simulink model "main"  (R2025b)
settings: Solver=FixedStepAuto  StartTime=0.0  StopTime=25  FixedStep=0.001  RelTol=1e-3
values from neighbouring files (symbols this model uses):
  Fin_MaxAngle = 8    [data.m]
  Physics_Gravity = -9.81    [data.m]
  Physics_SensorsNoiseFactor = 0.5    [data.m]
  PID_DCoeff = 50    [data.m]
  PID_DeadZone = 0.0    (= 0)    [data.m]
  PID_Kd = 50    [data.m]
  PID_Ki = 0    [data.m]
  PID_Kp = 400    [data.m]
  PID_SampleTime = 0.01    [data.m]
  PID_ServoDelay = 0.01    [data.m]
  PID_ServoMaxRate = 400    [data.m]
  Rocket_DesiredRotation = 90    [data.m]
libraries: simulink x5, simulink_extras x2, slpidlib x1, aerolibatmos2 x1, aerolibasang x1, aerolibnav x1, aerolibanim x1
settings Model: Creator=Filip  LastModifiedBy=Filip
settings SolverCC: EnableFixedStepZeroCrossing=on
settings RTWCC: GenCodeOnly=on
settings SimscapeCC: SimscapeLogDecimation=1  SimscapeLogDataHistory=5000

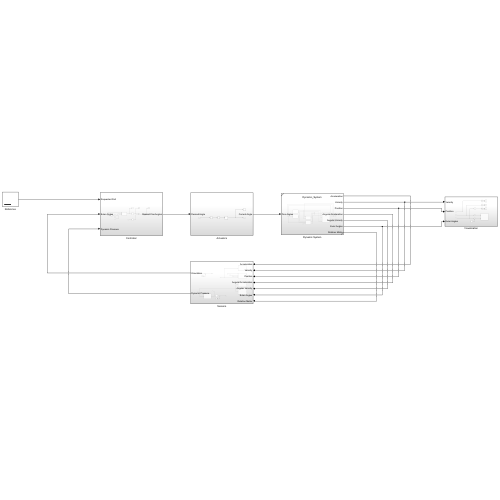
[thumbnail: Simulink's stored preview of the top-level diagram]
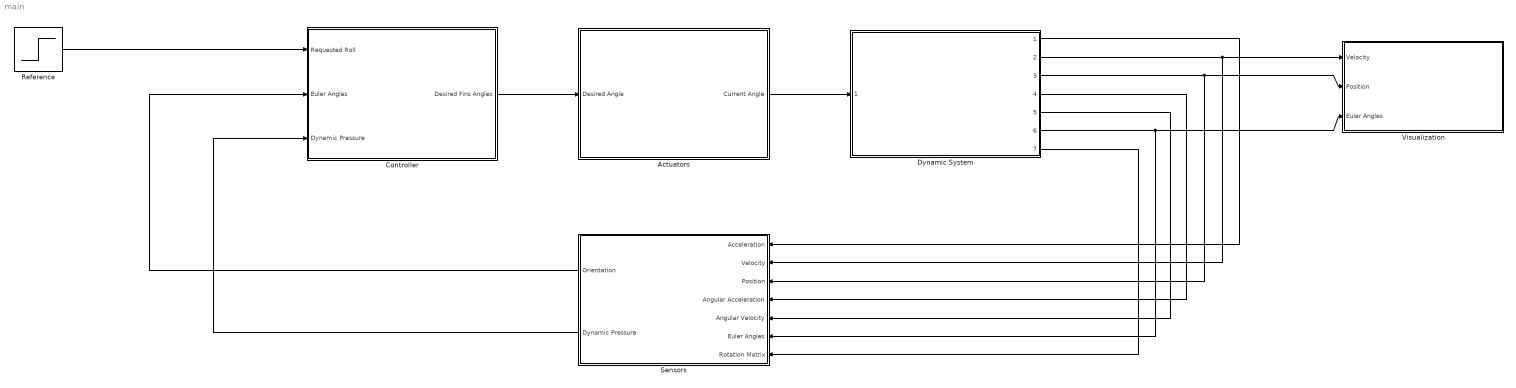
== system main ==
  Actuators : Subsystem
  Controller : Subsystem
  Dynamic System : Subsystem  ReferencedSubsystem=Dynamic_System
  Reference : Step  Time=2  After=Rocket_DesiredRotation  SampleTime=0
  Sensors : Subsystem
  Visualization : Subsystem
  wires:
  Controller/1(Desired Fins Angles) -> Actuators/1(Desired Angle)
  Actuators/1(Current Angle) -> Dynamic System/1
  Reference/1 -> Controller/1(Requested Roll)
  Dynamic System/2 -> Sensors/2(Velocity), Visualization/1(Velocity)
  Dynamic System/3 -> Sensors/3(Position), Visualization/2(Position)
  Dynamic System/6 -> Sensors/6(Euler Angles), Visualization/3(Euler Angles)
  Sensors/1(Orientation) -> Controller/2(Euler Angles)
  Sensors/2(Dynamic Pressure) -> Controller/3(Dynamic Pressure)
  Dynamic System/1 -> Sensors/1(Acceleration)
  Dynamic System/4 -> Sensors/4(Angular Acceleration)
  Dynamic System/5 -> Sensors/5(Angular Velocity)
  Dynamic System/7 -> Sensors/7(Rotation Matrix)

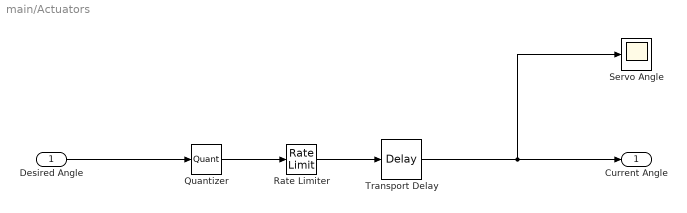
== system main/Actuators ==
  Desired Angle : Inport
  Quantizer : Quantizer  QuantizationInterval=PID_ServoStep
  Rate Limiter : RateLimiter  RisingSlewLimit=+PID_ServoMaxRate  FallingSlewLimit=-PID_ServoMaxRate  SampleTimeMode=inherited
  Servo Angle : Scope
      settings: DataLoggingVariableName=ScopeData2
  Transport Delay : TransportDelay  DelayTime=PID_ServoDelay
  Current Angle : Outport
  wires:
  Rate Limiter/1 -> Transport Delay/1
  Transport Delay/1 -> Servo Angle/1, Current Angle/1
  Quantizer/1 -> Rate Limiter/1
  Desired Angle/1 -> Quantizer/1

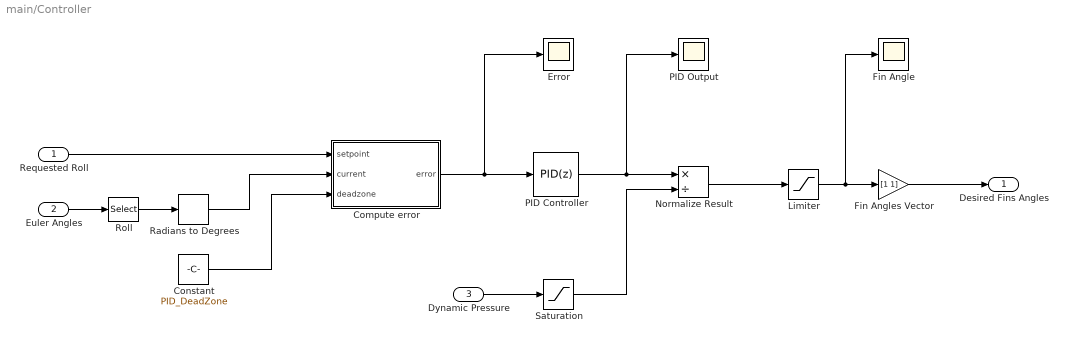
== system main/Controller ==
  Requested Roll : Inport
  Euler Angles : Inport  Port=2
  Dynamic Pressure : Inport  Port=3
  Compute error : MATLAB Function  TreatAsAtomicUnit=on
  Constant : Constant  Value=PID_DeadZone
  Error : Scope
      settings: ActiveDisplayYMinimum=-22.0959398024316  ActiveDisplayYMaximum=103.3390551975684
  Fin Angle : Scope
      settings: DataLoggingVariableName=ScopeData3
  Fin Angles Vector : Gain  Gain=[1 1]
  Limiter : Saturate  UpperLimit=+Fin_MaxAngle  LowerLimit=-Fin_MaxAngle
  Normalize Result : Product  Inputs=*/
  PID Controller : slpidlib/PID Controller  Controller=PID  Form=Parallel  TimeDomain=Discrete-time  UseExternalTs=off  SampleTime=PID_SampleTime  IntegratorMethod=Forward Euler  FilterMethod=Forward Euler  ControllerParametersSource=internal  P=PID_Kp  I=PID_Ki  UseKiTs=off  D=PID_Kd  UseExternalDerivativeSource=off  N=PID_DCoeff  UseFilter=on  TunerSelectOption=Transfer Function Based (PID Tuner App)  InitialConditionSource=internal  InitialConditionForIntegrator=0  InitialConditionForFilter=0  DifferentiatorICPrevScaledInput=0  ExternalReset=none  TrackingMode=off  Kt=1  LimitOutput=off  SatLimitsSource=internal  UpperSaturationLimit=inf  LowerSaturationLimit=-inf  LinearizeAsGain=on  AntiWindupMode=none  Kb=1  LimitIntegrator=off  UpperIntegratorSaturationLimit=inf  LowerIntegratorSaturationLimit=-inf  POutMin=[]  POutMax=[]  IOutMin=[]  IOutMax=[]  DOutMin=[]  DOutMax=[]  NOutMin=[]  NOutMax=[]  SumOutMin=[]  SumOutMax=[]  SaturationOutMin=[]  SaturationOutMax=[]  PParamMin=[]  PParamMax=[]  IParamMin=[]  IParamMax=[]  DParamMin=[]  DParamMax=[]  NParamMin=[]  NParamMax=[]  KbParamMin=[]  KbParamMax=[]  KtParamMin=[]  KtParamMax=[]  KbOutMin=[]  KbOutMax=[]  KtOutMin=[]  KtOutMax=[]  IntegratorOutMin=[]  IntegratorOutMax=[]  FilterOutMin=[]  FilterOutMax=[]  SumI1OutMin=[]  SumI1OutMax=[]  SumI2OutMin=[]  SumI2OutMax=[]  SumI3OutMin=[]  SumI3OutMax=[]  SumI4OutMin=[]  SumI4OutMax=[]  SumDOutMin=[]  SumDOutMax=[]  DifferentiatorOutMin=[]  DifferentiatorOutMax=[]  FilterDiffOutCoefMin=[]  FilterDiffOutCoefMax=[]  ReciprocalOutMin=[]  ReciprocalOutMax=[]  SumDenOutMin=[]  SumDenOutMax=[]  SumNumOutMin=[]  SumNumOutMax=[]  DivideOutMin=[]  DivideOutMax=[]  UdiffTsProdOutMin=[]  UdiffTsProdOutMax=[]  NTsProdOutMin=[]  NTsProdOutMax=[]  UintegralTsProdOutMin=[]  UintegralTsProdOutMax=[]  UngainTsProdOutMin=[]  UngainTsProdOutMax=[]  ClampingZeroOutDataTypeStr=Inherit: Inherit via back propagation  ClampingZeroOutMin=[]  ClampingZeroOutMax=[]  FilterDenConstantOutDataTypeStr=Inherit: Inherit via back propagation  FilterDenConstantOutMin=[]  FilterDenConstantOutMax=[]  PCopyOutDataTypeStr=Inherit: Inherit via back propagation  PCopyOutMin=[]  PCopyOutMax=[]  NCopyOutDataTypeStr=Inherit: Inherit via back propagation  NCopyOutMin=[]  NCopyOutMax=[]  IntegratorContinuousStateAttributes=''  IntegratorStateMustResolveToSignalObject=off  IntegratorRTWStateStorageClass=Auto  FilterContinuousStateAttributes=''  FilterStateMustResolveToSignalObject=off  FilterRTWStateStorageClass=Auto  ParallelPVariant=InternalParameters  IdealPVariant=Disabled  IVariant=InternalParameters  DVariant=InternalParameters  IntegratorVariant=Discrete  SatVariant=Disabled  AWVariant=Passthrough  PCopyVariant=Disabled  TRVariant=Disabled  FdbkBlocksVariant=Forward  IdealPFdbkVariant=Disabled  SatFdbkVariant=Disabled  DerivativeFilterVariant=ForwardEulerFilter  NVariant=InternalParameters  NCopyVariant=Disabled  FilterICVariant=InternalICsFilter  IntegratorICVariant=InternalICs  ExternalResetVariant=Disabled  TRSumVariant=Passthrough  SumFdbkVariant=Disabled  SumVariant=Sum_PID  TsampFilterVariant=InternalTs  TsampNgainVariant=Passthrough  TsampIntegralVariant=Disabled_SignalSpec  ExternalSaturationOutDataTypeStr=Inherit: Same as second input  DerivativeSourceVariant=ErrorSignal  PreIntVariant=InternalPreInt
  PID Output : Scope
      settings: ActiveDisplayYMinimum=-44847.41434  ActiveDisplayYMaximum=228488.88968
  Radians to Degrees : simulink_extras/Transformations/Radians to Degrees
  Roll : Selector  InputPortWidth=3  IndexOptions=Index vector (dialog)  Indices=[3]  OutputSizes=1
  Saturation : Saturate  UpperLimit=1000000  LowerLimit=10
  Desired Fins Angles : Outport
  wires:
  Euler Angles/1 -> Roll/1
  Requested Roll/1 -> Compute error/1(setpoint)
  Normalize Result/1 -> Limiter/1
  Limiter/1 -> Fin Angle/1, Fin Angles Vector/1
  Roll/1 -> Radians to Degrees/1
  Fin Angles Vector/1 -> Desired Fins Angles/1
  Dynamic Pressure/1 -> Saturation/1
  Saturation/1 -> Normalize Result/2
  Compute error/1(error) -> PID Controller/1, Error/1
  Radians to Degrees/1 -> Compute error/2(current)
  PID Controller/1 -> PID Output/1, Normalize Result/1
  Constant/1 -> Compute error/3(deadzone)

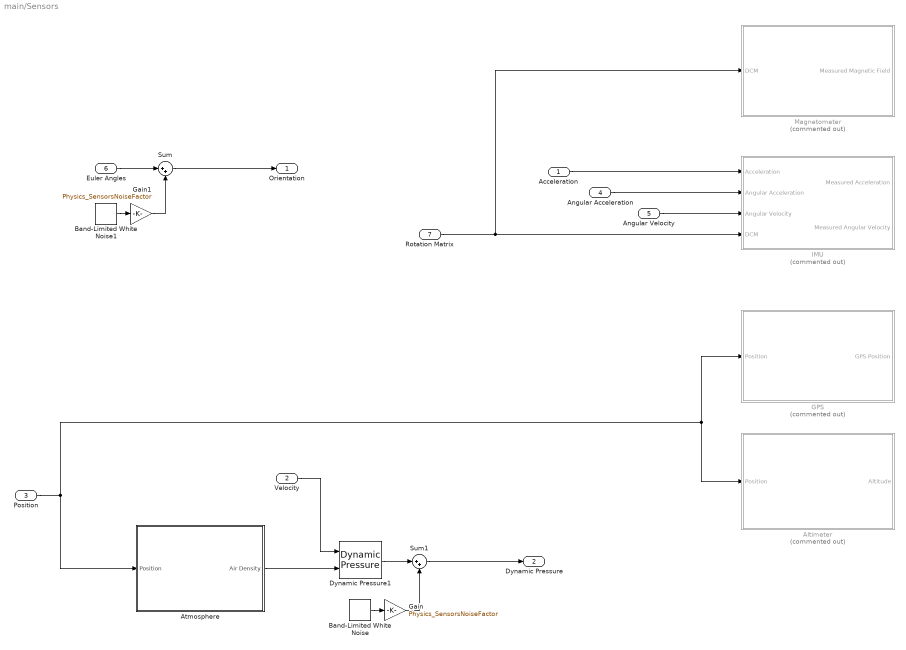
== system main/Sensors ==
  Acceleration : Inport
  Velocity : Inport  Port=2
  Position : Inport  Port=3
  Angular Acceleration : Inport  Port=4
  Angular Velocity : Inport  Port=5
  Euler Angles : Inport  Port=6
  Rotation Matrix : Inport  Port=7
  Altimeter : Subsystem  Commented=on
  Atmosphere : Subsystem
  Band-Limited White Noise : simulink/Sources/Band-Limited White Noise  Cov=[0.005]  Ts=0.002  seed=[23341]
  Band-Limited White Noise1 : simulink/Sources/Band-Limited White Noise  Cov=[0.0000005]  Ts=0.002  seed=[23341]
  Dynamic Pressure1 : aerolibasang/Dynamic Pressure
  GPS : Subsystem  Commented=on
  Gain : Gain  Gain=Physics_SensorsNoiseFactor
  Gain1 : Gain  Gain=Physics_SensorsNoiseFactor
  IMU : Subsystem  Commented=on
  Magnetometer : Subsystem  Commented=on
  Sum : Sum  Inputs=|++
  Sum1 : Sum  Inputs=|++
  Orientation : Outport
  Dynamic Pressure : Outport  Port=2
  wires:
  Position/1 -> GPS/1(Position), Altimeter/1(Position), Atmosphere/1(Position)
  Velocity/1 -> Dynamic Pressure1/1
  Atmosphere/1(Air Density) -> Dynamic Pressure1/2
  Rotation Matrix/1 -> Magnetometer/1(DCM), IMU/4(DCM)
  Acceleration/1 -> IMU/1(Acceleration)
  Angular Acceleration/1 -> IMU/2(Angular Acceleration)
  Angular Velocity/1 -> IMU/3(Angular Velocity)
  Euler Angles/1 -> Sum/1
  Sum/1 -> Orientation/1
  Dynamic Pressure1/1 -> Sum1/1
  Sum1/1 -> Dynamic Pressure/1
  Band-Limited White Noise/1 -> Gain/1
  Gain/1 -> Sum1/2
  Band-Limited White Noise1/1 -> Gain1/1
  Gain1/1 -> Sum/2

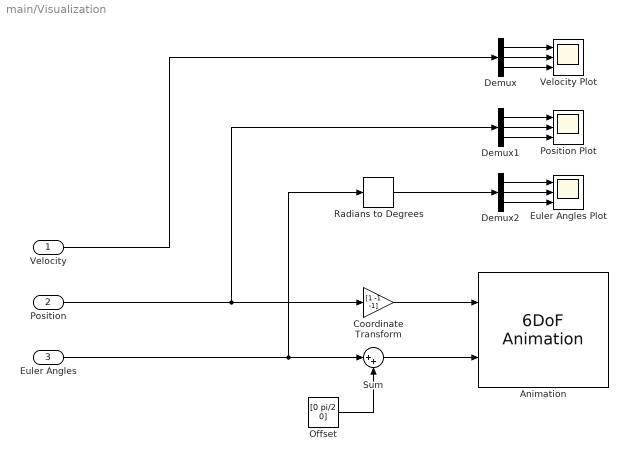
== system main/Visualization ==
  Velocity : Inport
  Position : Inport  Port=2
  Euler Angles : Inport  Port=3
  Animation : aerolibanim/6DoF Animation  u1=[-4000 4000 -4000 4000 -4000 4000]  u2=0.01  u3=5  u4=[0 0 0]  u5=Fly alongside  u6=[50 50 -50]  u7=10  u8=off
  Coordinate Transform : Gain  Gain=[1 -1 -1]
  Demux : Demux  Outputs=3
  Demux1 : Demux  Outputs=3
  Demux2 : Demux  Outputs=3
  Euler Angles Plot : Scope  NumInputPorts=3
      settings: ActiveDisplayYMinimum=-1  ActiveDisplayYMaximum=1  DataLoggingVariableName=ScopeData2
  Offset : Constant  Value=[0 pi/2 0]
  Position Plot : Scope  NumInputPorts=3
      settings: ActiveDisplayYMinimum=-1  ActiveDisplayYMaximum=1
  Radians to Degrees : simulink_extras/Transformations/Radians to Degrees
  Sum : Sum  Inputs=|++
  Velocity Plot : Scope  NumInputPorts=3
      settings: ActiveDisplayYMinimum=-1  ActiveDisplayYMaximum=1
  wires:
  Demux1/2 -> Position Plot/2
  Position/1 -> Coordinate Transform/1, Demux1/1
  Demux2/1 -> Euler Angles Plot/1
  Demux1/3 -> Position Plot/3
  Demux/2 -> Velocity Plot/2
  Demux1/1 -> Position Plot/1
  Demux/3 -> Velocity Plot/3
  Demux/1 -> Velocity Plot/1
  Demux2/2 -> Euler Angles Plot/2
  Demux2/3 -> Euler Angles Plot/3
  Velocity/1 -> Demux/1
  Radians to Degrees/1 -> Demux2/1
  Offset/1 -> Sum/2
  Euler Angles/1 -> Radians to Degrees/1, Sum/1
  Coordinate Transform/1 -> Animation/1
  Sum/1 -> Animation/2

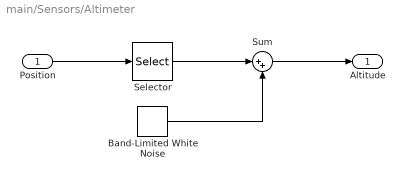
== system main/Sensors/Altimeter ==
  Position : Inport
  Band-Limited White Noise : simulink/Sources/Band-Limited White Noise  Cov=[0.00005]  Ts=0.002  seed=[23341]
  Selector : Selector  InputPortWidth=3  IndexOptions=Index vector (dialog)  Indices=[3]  OutputSizes=1
  Sum : Sum  Inputs=|++
  Altitude : Outport
  wires:
  Position/1 -> Selector/1
  Sum/1 -> Altitude/1
  Band-Limited White Noise/1 -> Sum/2
  Selector/1 -> Sum/1

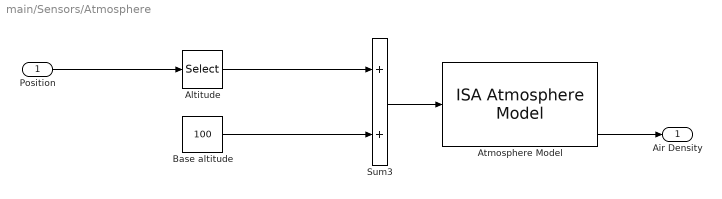
== system main/Sensors/Atmosphere ==
  Position : Inport
  Altitude : Selector  IndexMode=Zero-based  InputPortWidth=3  IndexOptions=Index vector (dialog)  Indices=2  OutputSizes=1
  Atmosphere Model : aerolibatmos2/ISA Atmosphere Model  useExtended=off  action=Warning  custom=off  viscosityOut=off  g=9.80665  gamma=1.4  R=287.0531  L=0.0065  h_trop=11000  h_strat=20000  rho0=1.225  P0=101325  T0=288.15  h0=0  S=110.4  Tref=273.15  muref=1.716e-5
  Base altitude : Constant  Value=100
  Sum3 : Sum
  Air Density : Outport
  wires:
  Atmosphere Model/4 -> Air Density/1
  Base altitude/1 -> Sum3/2
  Sum3/1 -> Atmosphere Model/1
  Position/1 -> Altitude/1
  Altitude/1 -> Sum3/1

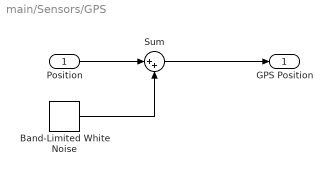
== system main/Sensors/GPS ==
  Position : Inport
  Band-Limited White Noise : simulink/Sources/Band-Limited White Noise  Cov=[0.1]  Ts=0.05  seed=[23341]
  Sum : Sum  Inputs=|++
  GPS Position : Outport
  wires:
  Sum/1 -> GPS Position/1
  Band-Limited White Noise/1 -> Sum/2
  Position/1 -> Sum/1

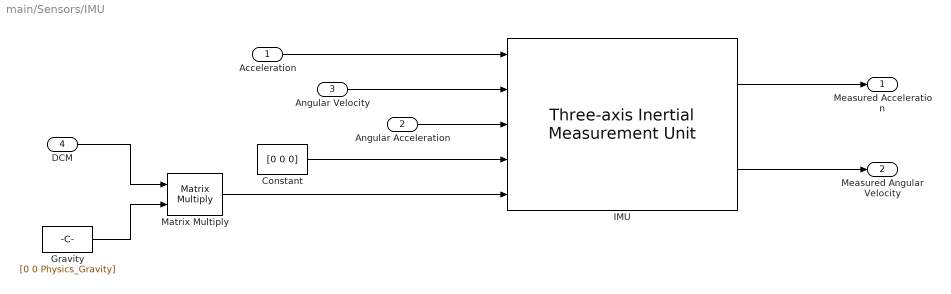
== system main/Sensors/IMU ==
  Acceleration : Inport
  Angular Acceleration : Inport  Port=2
  Angular Velocity : Inport  Port=3
  DCM : Inport  Port=4
  Constant : Constant  Value=[0 0 0]
  Gravity : Constant  Value=[0 0 Physics_Gravity]
  IMU : aerolibnav/Three-axis Inertial Measurement Unit  units=Metric (MKS)  imu=[0 0 0]  i_Ts=0.002  dtype_a=on  w_a=190  z_a=0.707  a_sf_cc=[1 0 0; 0 1 0; 0 0 1]  a_bias=[0 0 0]  a_sat="[-inf  -inf  -inf  inf inf inf]"  dtype_g=on  w_g=190  z_g=0.707  g_sf_cc=[1 0 0; 0 1 0; 0 0 1]  g_bias=[0 0 0]  g_sens=[0 0 0]  g_sat="[-inf  -inf  -inf  inf inf inf]"  i_rand=on  i_seeds=[23093 23094 23095 23096 23097 23098]  i_pow=[0.0002 0.0002 0.0002 0.000003 0.000003 0.000003]
  Matrix Multiply : Product  Multiplication=Matrix(*)
  Measured Acceleration : Outport
  Measured Angular Velocity : Outport  Port=2
  wires:
  IMU/1 -> Measured Acceleration/1
  Gravity/1 -> Matrix Multiply/2
  Matrix Multiply/1 -> IMU/5
  Acceleration/1 -> IMU/1
  DCM/1 -> Matrix Multiply/1
  Constant/1 -> IMU/4
  Angular Velocity/1 -> IMU/2
  Angular Acceleration/1 -> IMU/3
  IMU/2 -> Measured Angular Velocity/1

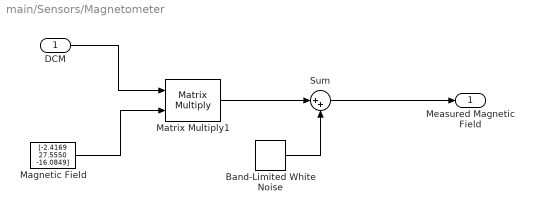
== system main/Sensors/Magnetometer ==
  DCM : Inport
  Band-Limited White Noise : simulink/Sources/Band-Limited White Noise  Cov=[0.001]  Ts=0.002  seed=[23341]
  Magnetic Field : Constant  Value=[-2.4169 27.5550 -16.0849]
  Matrix Multiply1 : Product  Multiplication=Matrix(*)
  Sum : Sum  Inputs=|++
  Measured Magnetic Field : Outport
  wires:
  Magnetic Field/1 -> Matrix Multiply1/2
  DCM/1 -> Matrix Multiply1/1
  Band-Limited White Noise/1 -> Sum/2
  Matrix Multiply1/1 -> Sum/1
  Sum/1 -> Measured Magnetic Field/1

== matlab function main/Controller/Compute error ==
  data: setpoint input; error output; current input; deadzone input
function error = fcn(setpoint, current, deadzone)

e1 = setpoint - current;

if e1 > 0
    e2 = e1 - 360;
else
    e2 = e1 + 360;
end

if abs(e1) < abs(e2)
    error = e1;
else
    error = e2;
end

if abs(error) <= deadzone
    error = 0;
end
